simulink model "LQRTrailerKinematics"  (R2018a)
settings: Solver=ode45  StartTime=0.0  StopTime=sim_time  FixedStep=.001  RelTol=1e-9
values from neighbouring files (symbols this model uses):
  A = [0 V ... (first row only)    [kinematicLQR_FF.m]    (also in trailerKinematicsLQR.m = [0       0         0)
  B = [0 ... (first row only)    [kinematicLQR_FF.m]    (also in trailerKinematicsLQR.m = [vr./lt)
  C = eye(2)    [kinematicLQR_FF.m]    (also in trailerKinematicsLQR.m = eye(3))
  ICs = [vehicleIC(2), deg2rad(45)]    [kinematicLQR_FF.m]    (also in trailerKinematicsLQR.m = [deg2rad(270); deg2rad(270); y_IC])
  L = 1.524    [kinematicLQR_FF.m]
  lh = -0.2286    [trailerKinematicsLQR.m]
  lr = 5.7336    [trailerKinematicsLQR.m]
  lt = 12.192    [trailerKinematicsLQR.m]
  tractorIC = [trailerIC(1), trailerIC(2) - (lt+lh)]    [trailerKinematicsLQR.m]
  trailerIC = [track_vector(1,1)-y_IC*sin(3*pi/2), track_vector(1, 2)+y_IC*cos(3*pi/2)]    [trailerKinematicsLQR.m]
  vr = -4.5    [trailerKinematicsLQR.m]
undefined symbols (not defined in the file or in its folder): K
settings Model: Creator=journ  LastModifiedBy=journeyman
settings SolverCC: ZeroCrossAlgorithm=Adaptive
settings OptimizationCC: LifeSpan=inf
settings DebuggingCC: MaxConsecutiveZCsMsg=none  SFExecutionAtInitializationDiag=none
settings CodeAppCC: StateflowObjectComments=on

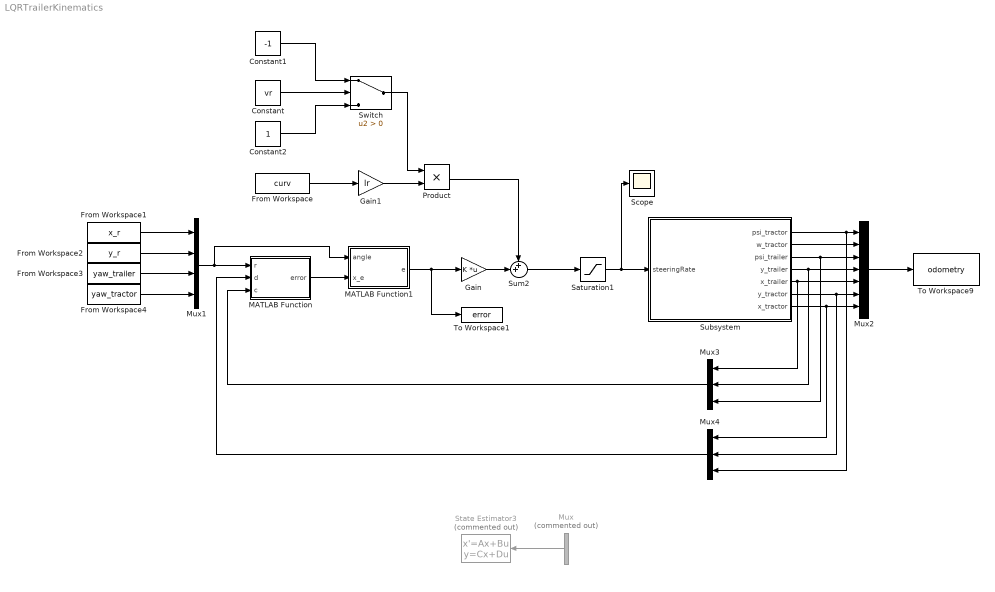
== system LQRTrailerKinematics ==
  Constant : Constant  Value=vr
  Constant1 : Constant  Value=-1
  Constant2 : Constant
  From Workspace : FromWorkspace  VariableName=curv  SampleTime=0
  From Workspace1 : FromWorkspace  VariableName=x_r  SampleTime=0  OutputAfterFinalValue=Holding final value
  From Workspace2 : FromWorkspace  VariableName=y_r  SampleTime=0
  From Workspace3 : FromWorkspace  VariableName=yaw_trailer  SampleTime=0
  From Workspace4 : FromWorkspace  VariableName=yaw_tractor  SampleTime=0
  Gain : Gain  Gain=K  Multiplication=Matrix(K*u)
  Gain1 : Gain  Gain=lr
  MATLAB Function : MATLAB Function  TreatAsAtomicUnit=on
  MATLAB Function1 : MATLAB Function  TreatAsAtomicUnit=on
  Mux : Mux  Commented=on  Inputs=2
  Mux1 : Mux
  Mux2 : Mux  Inputs=7
  Mux3 : Mux  Inputs=3
  Mux4 : Mux  Inputs=3
  Product : Product
  Saturation1 : Saturate  UpperLimit=deg2rad(30)  LowerLimit=-deg2rad(30)
  Scope : Scope
  State Estimator3 : StateSpace  Commented=on  A=A - L*C  B=[B L]  C=eye(4)  D=zeros(4,3)  InitialCondition=ICs
  Subsystem : Subsystem
  Sum2 : Sum  Inputs=++|
  Switch : Switch  Criteria=u2 > Threshold
  To Workspace1 : ToWorkspace  VariableName=error  SampleTime=-1
  To Workspace9 : ToWorkspace  VariableName=odometry  SampleTime=-1
  wires:
  Mux/1 -> State Estimator3/1
  From Workspace/1 -> Gain1/1
  Subsystem/1(psi_tractor) -> Mux4/3, Mux2/1
  Subsystem/2(w_tractor) -> Mux2/2
  Subsystem/4(y_trailer) -> Mux2/4, Mux3/2
  Subsystem/5(x_trailer) -> Mux2/5, Mux3/1
  Subsystem/6(y_tractor) -> Mux4/2, Mux2/6
  Subsystem/7(x_tractor) -> Mux4/1, Mux2/7
  Mux2/1 -> To Workspace9/1
  MATLAB Function1/1(e) -> Gain/1, To Workspace1/1
  Mux1/1 -> MATLAB Function1/1(angle), MATLAB Function/1(r)
  From Workspace3/1 -> Mux1/3
  From Workspace2/1 -> Mux1/2
  From Workspace1/1 -> Mux1/1
  From Workspace4/1 -> Mux1/4
  Mux3/1 -> MATLAB Function/3(c)
  MATLAB Function/1(error) -> MATLAB Function1/2(x_e)
  Gain1/1 -> Product/2
  Saturation1/1 -> Scope/1, Subsystem/1(steeringRate)
  Mux4/1 -> MATLAB Function/2(d)
  Subsystem/3(psi_trailer) -> Mux3/3, Mux2/3
  Sum2/1 -> Saturation1/1
  Gain/1 -> Sum2/2
  Product/1 -> Sum2/1
  Constant/1 -> Switch/2
  Switch/1 -> Product/1
  Constant2/1 -> Switch/3
  Constant1/1 -> Switch/1

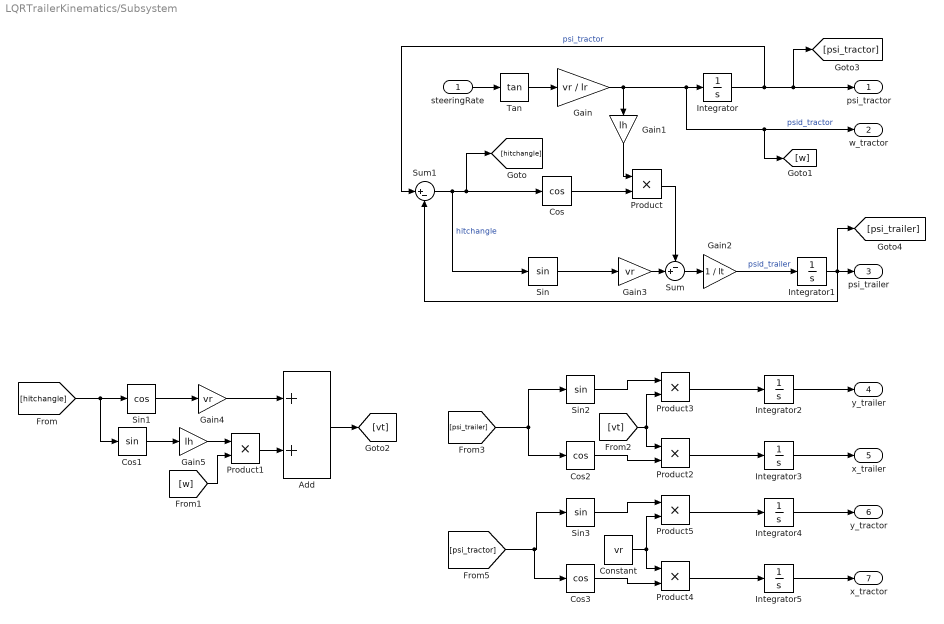
== system LQRTrailerKinematics/Subsystem ==
  steeringRate : Inport
  Add : Sum
  Constant : Constant  Value=vr
  Cos : Trigonometry  Operator=cos
  Cos1 : Trigonometry
  Cos2 : Trigonometry  Operator=cos
  Cos3 : Trigonometry  Operator=cos
  Gain : Gain  Gain=vr / lr
  Gain1 : Gain  Gain=lh
  Gain2 : Gain  Gain=1 / lt
  Gain3 : Gain  Gain=vr
  Gain4 : Gain  Gain=vr
  Gain5 : Gain  Gain=lh
  Integrator : Integrator  InitialCondition=ICs(1)
  Integrator1 : Integrator  InitialCondition=ICs(2)
  Integrator2 : Integrator  InitialCondition=trailerIC(2)
  Integrator3 : Integrator  InitialCondition=trailerIC(1)
  Integrator4 : Integrator  InitialCondition=tractorIC(2)
  Integrator5 : Integrator  InitialCondition=tractorIC(1)
  Product{,1..5} (6 alike) : Product
  Sin : Trigonometry
  Sin1 : Trigonometry  Operator=cos
  Sin2 : Trigonometry
  Sin3 : Trigonometry
  Sum : Sum  Inputs=-+|
  Sum1 : Sum  Inputs=|+-
  Tan : Trigonometry  Operator=tan
  psi_tractor : Outport
  w_tractor : Outport  Port=2
  psi_trailer : Outport  Port=3
  y_trailer : Outport  Port=4
  x_trailer : Outport  Port=5
  y_tractor : Outport  Port=6
  x_tractor : Outport  Port=7
  wires:
  steeringRate/1 -> Tan/1
  Tan/1 -> Gain/1
  Gain/1 -> [w], w_tractor/1, Integrator/1, Gain1/1  "psid_tractor"
  Integrator/1 -> Sum1/1, [psi_tractor], psi_tractor/1  "psi_tractor"
  Sum/1 -> Gain2/1
  Gain1/1 -> Product/1
  Product/1 -> Sum/1
  Sum1/1 -> Sin/1, [hitchangle], Cos/1  "hitchangle"
  Cos/1 -> Product/2
  Sin/1 -> Gain3/1
  Gain3/1 -> Sum/2
  Gain2/1 -> Integrator1/1  "psid_trailer"
  Integrator1/1 -> [psi_trailer], Sum1/2, psi_trailer/1
  Sin1/1 -> Gain4/1
  Gain4/1 -> Add/1
  [hitchangle] -> Cos1/1, Sin1/1
  Cos1/1 -> Gain5/1
  Gain5/1 -> Product1/1
  Product1/1 -> Add/2
  [w] -> Product1/2
  Add/1 -> [vt]
  Cos2/1 -> Product2/2
  [vt] -> Product2/1, Product3/2
  Product2/1 -> Integrator3/1
  Product3/1 -> Integrator2/1
  Sin2/1 -> Product3/1
  [psi_trailer] -> Cos2/1, Sin2/1
  Sin3/1 -> Product5/1
  Product4/1 -> Integrator5/1
  Constant/1 -> Product4/1, Product5/2
  Cos3/1 -> Product4/2
  Product5/1 -> Integrator4/1
  [psi_tractor] -> Cos3/1, Sin3/1
  Integrator2/1 -> y_trailer/1
  Integrator3/1 -> x_trailer/1
  Integrator4/1 -> y_tractor/1
  Integrator5/1 -> x_tractor/1

== matlab function LQRTrailerKinematics/MATLAB Function1 ==
  data: angle input; e output; x_e input
function e = DCM(angle, x_e)
    % x_e = [x_r, y_r, yaw_trailer, yaw_tractor]
    e = zeros(3, 1);
    
    DCM = @(ang) [cos(ang)  sin(ang) 0;
                  -sin(ang) cos(ang) 0;
                  0         0        1];

    E = DCM(angle(3)) * x_e(1:3, 1);
    % e = [yaw_tractor, yaw_trailer, y_r]
    e(1, 1) = x_e(4, 1);
    e(2, 1) = E(3, 1);
    e(3, 1) = E(2, 1);

== matlab function LQRTrailerKinematics/MATLAB Function ==
  data: r input; d input; error output; c input
function error = safeminus(r, d, c)
    error = zeros(4, 1);
    error(1, 1) = r(1) - c(1);
    error(2, 1) = r(2) - c(2);
    
    cross = cos(c(3))*sin(r(3)) - sin(c(3))*cos(r(3));
    dot = cos(c(3))*cos(r(3)) + sin(c(3))*sin(r(3));
    error(3, 1) = atan2(cross, dot);
   
    cross_d = cos(d(3))*sin(r(3)) - sin(d(3))*cos(r(3));
    dot_d = cos(d(3))*cos(r(3)) + sin(d(3))*sin(r(3));
    error(4, 1) = atan2(cross_d, dot_d);
    
    % error = [x_e, y_e, yaw_trailer, yaw_tractor]
